simulink model "speed_profile"  (R2023a)
settings: Solver=VariableStepAuto  StartTime=0.0  StopTime=1477  RelTol=1e-3
libraries: autolibshared x1
settings Model: Creator=antaeug  LastModifiedBy=antaeug

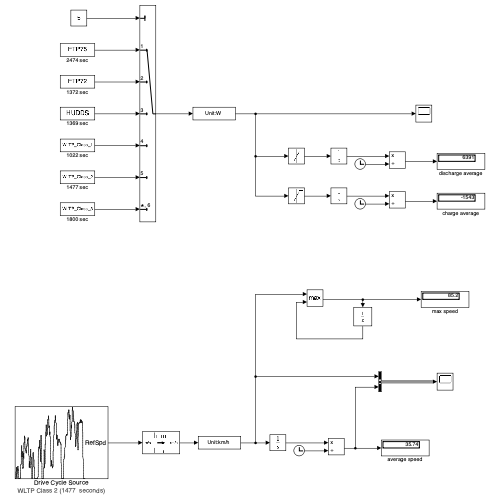
[thumbnail: Simulink's stored preview of the top-level diagram]
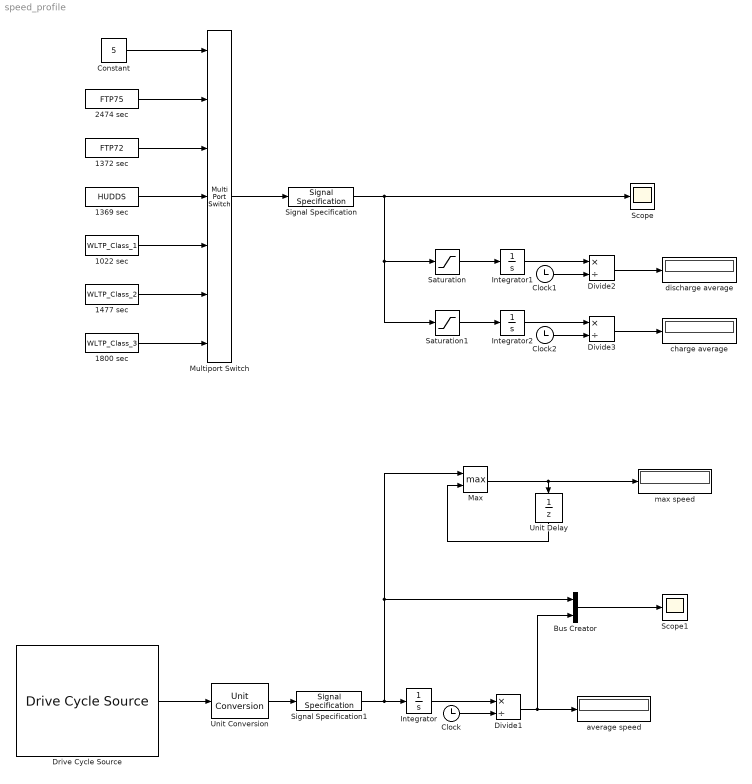
== system speed_profile ==
  1022 sec : FromWorkspace  VariableName=WLTP_Class_1  Interpolate=off  ZeroCross=off  OutputAfterFinalValue=Setting to zero
  1369 sec : FromWorkspace  VariableName=HUDDS  Interpolate=off  ZeroCross=off  OutputAfterFinalValue=Setting to zero
  1372 sec : FromWorkspace  VariableName=FTP72  Interpolate=off  ZeroCross=off  OutputAfterFinalValue=Setting to zero
  1477 sec : FromWorkspace  VariableName=WLTP_Class_2  Interpolate=off  ZeroCross=off  OutputAfterFinalValue=Setting to zero
  1800 sec : FromWorkspace  VariableName=WLTP_Class_3  Interpolate=off  ZeroCross=off  OutputAfterFinalValue=Setting to zero
  2474 sec : FromWorkspace  VariableName=FTP75  Interpolate=off  ZeroCross=off  OutputAfterFinalValue=Setting to zero
  Bus Creator : BusCreator  Inputs=2
  Clock : Clock
  Clock1 : Clock
  Clock2 : Clock
  Constant : Constant  Value=5
  Divide1 : Product  Inputs=*/
  Divide2 : Product  Inputs=*/
  Divide3 : Product  Inputs=*/
  Drive Cycle Source : autolibshared/Drive Cycle Source  cycleVar=WLTP Class 2  fileVar=cycleFTP75.mat  tfinal="1477  seconds"  cycleRepeat=off  outAccPort=off  outGearPort=off  gearList=No gear data  t_wot1=5  xdot_woto=0  xdot_wot1=30  t_wot2=20  xdot_wot2=0  t_wotend=30  srcUnit=m/s  outUnit=m/s  srcAccUnit=m/s/s  outAccUnit=m/s^2  dt=0  aMode=1  faultOption=off  velBnd=2  velBndUnit=mph  inUnit=m/s  timeBnd=1  failOption=off  stopSim=off  maxFaultCnt=10  maxFaultTime=2  maxTotFaultTime=15  traceOption=off  dtTrace=1  traceWindow=10  lastDCname=WLTP Class 3  lastOutUnit=mph  lastDT=0  lastTB=1  lastSB=2  forceCalcBound=off
  Integrator : Integrator
  Integrator1 : Integrator
  Integrator2 : Integrator
  Max : MinMax  Function=max  Inputs=2
  Multiport Switch : MultiPortSwitch  Inputs=6  SaturateOnIntegerOverflow=off  InputSameDT=off
  Saturation : Saturate  UpperLimit=200000  LowerLimit=0
  Saturation1 : Saturate  UpperLimit=0  LowerLimit=-200000
  Scope : Scope
  Scope1 : Scope
  Signal Specification : SignalSpecification  Unit=W
  Signal Specification1 : SignalSpecification  Unit=km/h
  Unit Conversion : UnitConversion
  Unit Delay : UnitDelay  SampleTime=-1  HasFrameUpgradeWarning=on
  average speed : Display
  charge average : Display
  discharge average : Display
  max speed : Display
  wires:
  Multiport Switch/1 -> Signal Specification/1
  1800 sec/1 -> Multiport Switch/7
  1369 sec/1 -> Multiport Switch/4
  1022 sec/1 -> Multiport Switch/5
  1372 sec/1 -> Multiport Switch/3
  1477 sec/1 -> Multiport Switch/6
  Constant/1 -> Multiport Switch/1
  2474 sec/1 -> Multiport Switch/2
  Signal Specification/1 -> Scope/1, Saturation1/1, Saturation/1
  Unit Conversion/1 -> Signal Specification1/1
  Drive Cycle Source/1 -> Unit Conversion/1
  Clock/1 -> Divide1/2
  Integrator/1 -> Divide1/1
  Signal Specification1/1 -> Max/1, Bus Creator/1, Integrator/1
  Divide1/1 -> Bus Creator/2, average speed/1
  Bus Creator/1 -> Scope1/1
  Clock1/1 -> Divide2/2
  Integrator1/1 -> Divide2/1
  Saturation/1 -> Integrator1/1
  Divide2/1 -> discharge average/1
  Saturation1/1 -> Integrator2/1
  Integrator2/1 -> Divide3/1
  Clock2/1 -> Divide3/2
  Divide3/1 -> charge average/1
  Max/1 -> max speed/1, Unit Delay/1
  Unit Delay/1 -> Max/2
